simulink model "modele_powertrain"  (R2025b)
settings: Solver=VariableStepAuto  StartTime=0.0  StopTime=20  RelTol=1e-3
values from neighbouring files (symbols this model uses):
  B = 1/eta_m    (= 2.5)    [variables_procom.m]
  Jprop = Jm/Rm^2    (= 18.6702)    [variables_procom.m]
  Kim = 23.2    [variables_procom.m]
  Kpm = 17.7    [variables_procom.m]
  Pe = 5    [variables_procom.m]
  Py = 60    [variables_procom.m]
  Rm = 1/2.9    (= 0.344827586207)    [variables_procom.m]
  tau_f = 0.2    [variables_procom.m]
libraries: slpidlib x1
settings Model: Creator=leagr  LastModifiedBy=f23berge

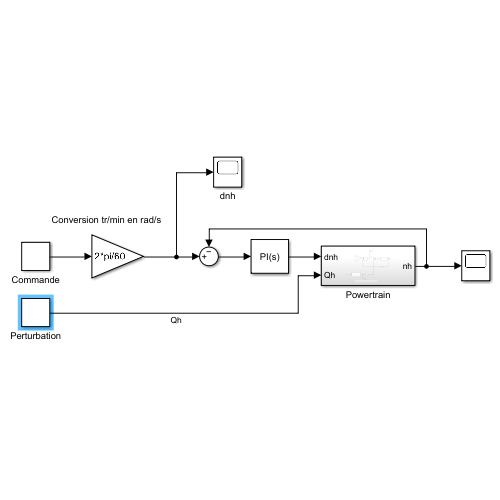
[thumbnail: Simulink's stored preview of the top-level diagram]
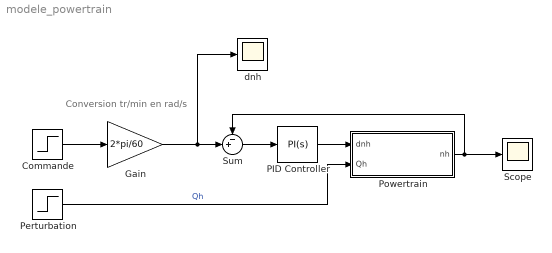
== system modele_powertrain ==
  note: Conversion tr/min en rad/s
  Commande : Step  After=750  SampleTime=0
  Gain : Gain  Gain=2*pi/60
  PID Controller : slpidlib/PID Controller  Controller=PI  Form=Parallel  TimeDomain=Continuous-time  UseExternalTs=off  SampleTime=-1  IntegratorMethod=Forward Euler  FilterMethod=Forward Euler  ControllerParametersSource=internal  P=Kpm  I=Kim  UseKiTs=off  D=0  UseExternalDerivativeSource=off  N=100  UseFilter=on  TunerSelectOption=Transfer Function Based (PID Tuner App)  InitialConditionSource=internal  InitialConditionForIntegrator=0  InitialConditionForFilter=0  DifferentiatorICPrevScaledInput=0  ExternalReset=none  TrackingMode=off  Kt=1  LimitOutput=off  SatLimitsSource=internal  UpperSaturationLimit=inf  LowerSaturationLimit=-inf  LinearizeAsGain=on  AntiWindupMode=none  Kb=1  LimitIntegrator=off  UpperIntegratorSaturationLimit=inf  LowerIntegratorSaturationLimit=-inf  POutMin=[]  POutMax=[]  IOutMin=[]  IOutMax=[]  DOutMin=[]  DOutMax=[]  NOutMin=[]  NOutMax=[]  SumOutMin=[]  SumOutMax=[]  SaturationOutMin=[]  SaturationOutMax=[]  PParamMin=[]  PParamMax=[]  IParamMin=[]  IParamMax=[]  DParamMin=[]  DParamMax=[]  NParamMin=[]  NParamMax=[]  KbParamMin=[]  KbParamMax=[]  KtParamMin=[]  KtParamMax=[]  KbOutMin=[]  KbOutMax=[]  KtOutMin=[]  KtOutMax=[]  IntegratorOutMin=[]  IntegratorOutMax=[]  FilterOutMin=[]  FilterOutMax=[]  SumI1OutMin=[]  SumI1OutMax=[]  SumI2OutMin=[]  SumI2OutMax=[]  SumI3OutMin=[]  SumI3OutMax=[]  SumI4OutMin=[]  SumI4OutMax=[]  SumDOutMin=[]  SumDOutMax=[]  DifferentiatorOutMin=[]  DifferentiatorOutMax=[]  FilterDiffOutCoefMin=[]  FilterDiffOutCoefMax=[]  ReciprocalOutMin=[]  ReciprocalOutMax=[]  SumDenOutMin=[]  SumDenOutMax=[]  SumNumOutMin=[]  SumNumOutMax=[]  DivideOutMin=[]  DivideOutMax=[]  UdiffTsProdOutMin=[]  UdiffTsProdOutMax=[]  NTsProdOutMin=[]  NTsProdOutMax=[]  UintegralTsProdOutMin=[]  UintegralTsProdOutMax=[]  UngainTsProdOutMin=[]  UngainTsProdOutMax=[]  ClampingZeroOutDataTypeStr=Inherit: Inherit via back propagation  ClampingZeroOutMin=[]  ClampingZeroOutMax=[]  FilterDenConstantOutDataTypeStr=Inherit: Inherit via back propagation  FilterDenConstantOutMin=[]  FilterDenConstantOutMax=[]  PCopyOutDataTypeStr=Inherit: Inherit via back propagation  PCopyOutMin=[]  PCopyOutMax=[]  NCopyOutDataTypeStr=Inherit: Inherit via back propagation  NCopyOutMin=[]  NCopyOutMax=[]  IntegratorContinuousStateAttributes=''  IntegratorStateMustResolveToSignalObject=off  IntegratorRTWStateStorageClass=Auto  FilterContinuousStateAttributes=''  FilterStateMustResolveToSignalObject=off  FilterRTWStateStorageClass=Auto  ParallelPVariant=InternalParameters  IdealPVariant=Disabled  IVariant=InternalParameters  DVariant=Disabled  IntegratorVariant=Continuous  SatVariant=Disabled  AWVariant=Passthrough  PCopyVariant=Disabled  TRVariant=Disabled  FdbkBlocksVariant=Forward  IdealPFdbkVariant=Disabled  SatFdbkVariant=Disabled  DerivativeFilterVariant=Disabled  NVariant=Disabled  NCopyVariant=Disabled_SignalSpec  FilterICVariant=Disabled  IntegratorICVariant=InternalICs  ExternalResetVariant=Disabled  TRSumVariant=Passthrough  SumFdbkVariant=Disabled  SumVariant=Sum_PI  TsampFilterVariant=InternalTs  TsampNgainVariant=Passthrough  TsampIntegralVariant=Disabled_SignalSpec  ExternalSaturationOutDataTypeStr=Inherit: Same as second input  DerivativeSourceVariant=Disabled  PreIntVariant=InternalPreInt
  Perturbation : Step  Time=10  After=500  SampleTime=0
  Powertrain : Subsystem
  Scope : Scope
      settings: ActiveDisplayYMinimum=-13.640525282609209  ActiveDisplayYMaximum=122.76472754348292
  Sum : Sum  Inputs=-+|
  dnh : Scope
      settings: ActiveDisplayYMinimum=-1  ActiveDisplayYMaximum=1  DataLoggingVariableName=ScopeData3
  wires:
  Perturbation/1 -> Powertrain/2(Qh)  "Qh"
  Powertrain/1(nh) -> Scope/1, Sum/1
  Commande/1 -> Gain/1
  Sum/1 -> PID Controller/1
  PID Controller/1 -> Powertrain/1(dnh)
  Gain/1 -> dnh/1, Sum/2

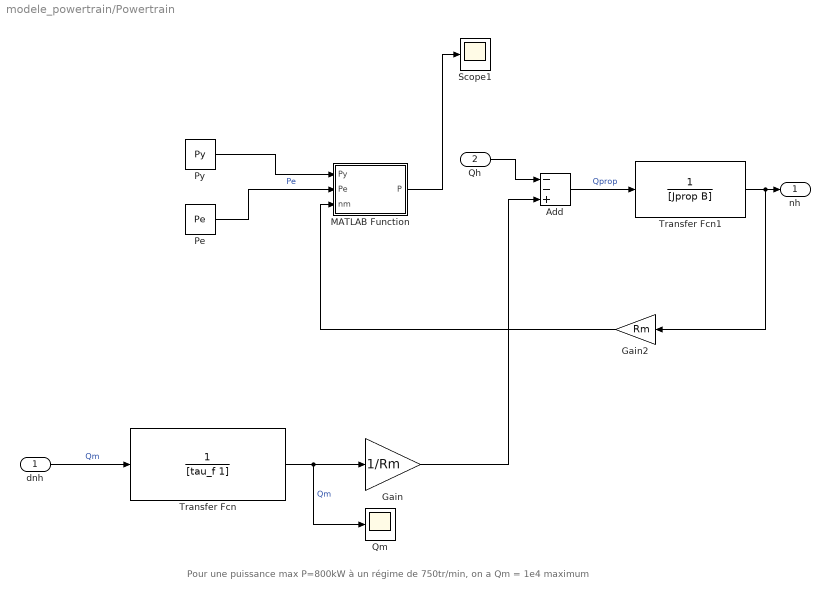
== system modele_powertrain/Powertrain ==
  note: Pour une puissance max P=800kW à un régime de 750tr/min, on a Qm = 1e4 maximum
  dnh : Inport
  Qh : Inport  Port=2
  Add : Sum  Inputs=--+
  Gain : Gain  Gain=1/Rm
  Gain2 : Gain  Gain=Rm
  MATLAB Function : MATLAB Function  TreatAsAtomicUnit=on
  Pe : Constant  Value=Pe
  Py : Constant  Value=Py
  Qm : Scope
      settings: ActiveDisplayYMinimum=-344.42934442499092  ActiveDisplayYMaximum=1247.8107231099157
  Scope1 : Scope
      settings: ActiveDisplayYMinimum=-1  ActiveDisplayYMaximum=1  DataLoggingVariableName=ScopeData2
  Transfer Fcn : TransferFcn  Denominator=[tau_f 1]
  Transfer Fcn1 : TransferFcn  Denominator=[Jprop B]
  nh : Outport
  wires:
  Qh/1 -> Add/1
  Add/1 -> Transfer Fcn1/1  "Qprop"
  Transfer Fcn1/1 -> Gain2/1, nh/1
  Gain/1 -> Add/3
  Transfer Fcn/1 -> Qm/1, Gain/1  "Qm"
  dnh/1 -> Transfer Fcn/1  "Qm"
  Gain2/1 -> MATLAB Function/3(nm)
  Py/1 -> MATLAB Function/1(Py)
  Pe/1 -> MATLAB Function/2(Pe)  "Pe"
  MATLAB Function/1(P) -> Scope1/1

== matlab function modele_powertrain/Powertrain/MATLAB Function ==
  data: Py input; P output; Pe input; nm input
function P = fcn(Py, Pe, nm)
threshold = 100*2*pi/60; % On ne branche l'aternateur et les pompes qu'une fois
                 % un certain régime atteint.
eta_p = 0.5;
    if nm < threshold
        P = 0;
    else
        P = (Pe*eta_p+Py)/nm;
    end
